simulink model "elorecsatolt"  (R2018a)
settings: Solver=VariableStepAuto  StartTime=0.0  StopTime=20  RelTol=1e-3
settings Model: Creator=Turing  LastModifiedBy=alfac

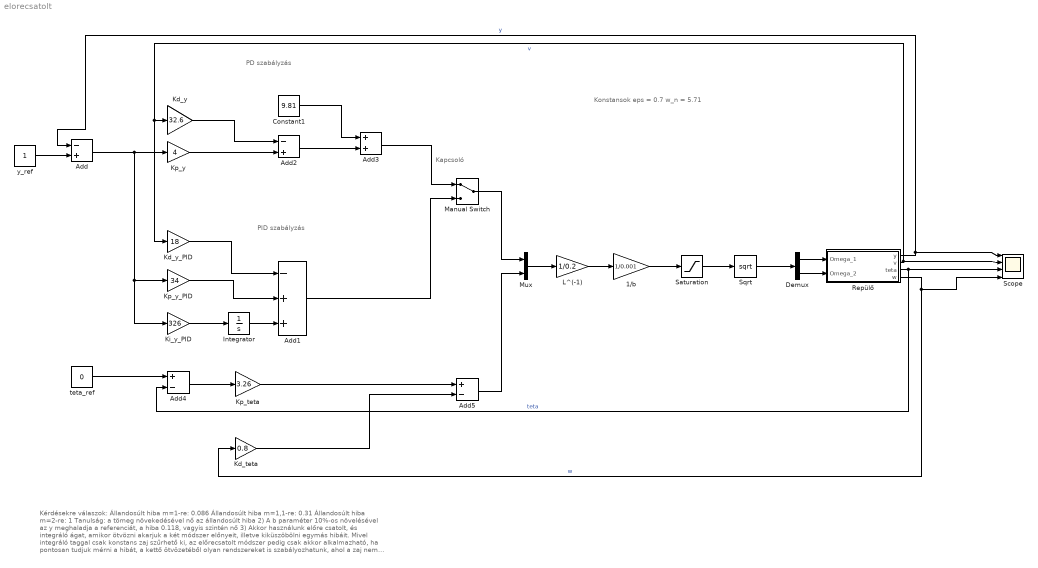
== system elorecsatolt ==
  note: PD szabályzás
  note: PID szabályzás
  note: Kapcsoló
  note: Konstansok
      |
      | eps = 0.7
      | w_n = 5.71
  note: Kérdésekre válaszok:
      | Állandosúlt hiba m=1-re: 0.086
      | Állandosúlt hiba m=1,1-re: 0.31
      | Állandosúlt hiba m=2-re: 1
      | Tanulság: a tömeg növekedésével nő az állandosúlt hiba
      | 2) A b paraméter 10%-os növelésével az y meghaladja a referenciát, a hiba 0.118, vagyis szintén nő
      | 3) Akkor használunk előre csatolt, és integráló ágat, amikor ötvözni akarjuk a két módszer előnyeit, illetve kiküszöbölni egymás hibáit. Mivel integráló taggal csak konstans zaj szűrhető
      | ki, az előrecsatolt módszer pedig csak akkor alkalmazható, ha pontosan tudjuk mérni a hibát, a kettő ötvözetéből olyan rendszereket is szabályozhatunk, ahol a zaj nem teljesen konstas
      | , illetve, nem pontosan mérhető.
  1/b : Gain  Gain=1/0.001
  Add : Sum  Inputs=-+
  Add1 : Sum  Inputs=-++
  Add2 : Sum  Inputs=-+
  Add3 : Sum
  Add4 : Sum  Inputs=+-
  Add5 : Sum  Inputs=+-
  Constant1 : Constant  Value=9.81
  Demux : Demux  Outputs=2
  Integrator : Integrator
  Kd_teta : Gain  Gain=0.8
  Kd_y : Gain  Gain=32.6
  Kd_y_PID : Gain  Gain=18
  Ki_y_PID : Gain  Gain=326
  Kp_teta : Gain  Gain=3.26
  Kp_y : Gain  Gain=4
  Kp_y_PID : Gain  Gain=34
  L^(-1) : Gain  Gain=1/0.2
  Manual Switch : ManualSwitch
  Mux : Mux  Inputs=2
  Repülő : Subsystem  mask{m=1, b=0.00110}
  Saturation : Saturate  UpperLimit=inf  LowerLimit=0
  Scope : Scope  NumInputPorts=4
  Sqrt : Sqrt  SaturateOnIntegerOverflow=on
  teta_ref : Constant  Value=0
  y_ref : Constant
  wires:
  y_ref/1 -> Add/2
  Add/1 -> Ki_y_PID/1, Kp_y_PID/1, Kp_y/1
  Ki_y_PID/1 -> Integrator/1
  Integrator/1 -> Add1/3
  Kd_y_PID/1 -> Add1/1
  Kp_y_PID/1 -> Add1/2
  Kp_y/1 -> Add2/2
  Kd_y/1 -> Add2/1
  Add2/1 -> Add3/2
  Constant1/1 -> Add3/1
  Add1/1 -> Manual Switch/2
  Add3/1 -> Manual Switch/1
  teta_ref/1 -> Add4/1
  Add4/1 -> Kp_teta/1
  Kp_teta/1 -> Add5/1
  Kd_teta/1 -> Add5/2
  Manual Switch/1 -> Mux/1
  Add5/1 -> Mux/2
  Mux/1 -> L^(-1)/1
  L^(-1)/1 -> 1/b/1
  1/b/1 -> Saturation/1
  Saturation/1 -> Sqrt/1
  Sqrt/1 -> Demux/1
  Demux/1 -> Repülő/1(Omega_1)
  Demux/2 -> Repülő/2(Omega_2)
  Repülő/3(teta) -> Scope/3, Add4/2  "teta"
  Repülő/4(w) -> Scope/4, Kd_teta/1  "w"
  Repülő/2(v) -> Scope/2, Kd_y_PID/1, Kd_y/1  "v"
  Repülő/1(y) -> Scope/1, Add/1  "y"

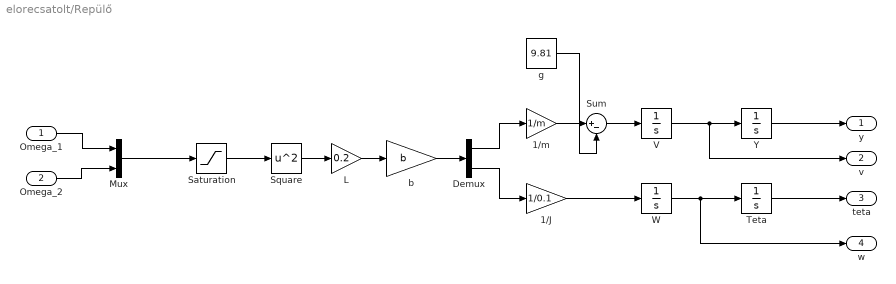
== system elorecsatolt/Repülő ==
  Omega_1 : Inport
  Omega_2 : Inport  Port=2
  "1/J " : Gain  Gain=1/0.1
  1/m : Gain  Gain=1/m
  Demux : Demux  Outputs=2
  L : Gain  Gain=0.2
  Mux : Mux  Inputs=2
  Saturation : Saturate  UpperLimit=inf  LowerLimit=0
  Square : Math  Operator=square  SaturateOnIntegerOverflow=on
  Sum : Sum  Inputs=|+-
  Teta : Integrator
  V : Integrator
  W : Integrator
  Y : Integrator
  b : Gain  Gain=b
  g : Constant  Value=9.81
  y : Outport
  v : Outport  Port=2
  teta : Outport  Port=3
  w : Outport  Port=4
  wires:
  Omega_2/1 -> Mux/2
  Omega_1/1 -> Mux/1
  Mux/1 -> Saturation/1
  Saturation/1 -> Square/1
  Square/1 -> L/1
  L/1 -> b/1
  b/1 -> Demux/1
  Demux/2 -> "1/J "/1
  Demux/1 -> 1/m/1
  g/1 -> Sum/2
  1/m/1 -> Sum/1
  Sum/1 -> V/1
  "1/J "/1 -> W/1
  W/1 -> w/1, Teta/1
  V/1 -> v/1, Y/1
  Y/1 -> y/1
  Teta/1 -> teta/1
